simulink model "p4_system_arch_master"  (R2020a)
settings: Solver=VariableStepAuto  StartTime=0.0  StopTime=10.0  RelTol=1e-3
(part 4 of 11)

== system p4_system_arch_master/System 2 : Gearbox System/2.1 Torque Multiplication System/2.1.3 Gearset System 3 ==
  2.1.3.0.1 Pinion : ModelReference  ModelNameDialog=GearsetPinion  SimulationMode=Normal  ModelReferenceVersion=1.1
      settings: PortSchema="{\"entries\":[{\"content\":{\"headerSize\":38,\"margin\":15,\"minimumSpacing\":25,\"sides\":[{\"content\":{\"connectorIds\":[]},\"type\":\"ConnectorPlacement.EquallySpacedRectSide\",\"uuid\":\"a1de0a4a-4383-4256-97c8-b4b7017d79c3\"},{\"content\":{\"connectorIds\":[],\"side\":\"RIGHT\"},\"type\":\"ConnectorPlacement.EquallySpacedRectSide\",\"uuid\":\"b959f0e1-b665-4773-a9ab-23b80a79bba3\"},{\"content\":{\"connectorIds\":[],\"side\":\"TOP\"},\"type\":\"ConnectorPlacement.EquallySpacedRectSide\",\"uuid\":\"884e98bd-fa8a-4556-86a7-182eb6de8f96\"}]},\"type\":\"ConnectorPlacement.EquallySpacedConnector\",\"uuid\":\"31d5ce3f-6fbe-45a5-a872-1e90bd0aea01\"}],\"packageUris\":[\"http://schema.mathworks.com/mf0/Connector/19700101\"],\"version\":\"1.0\"}"
  2.1.3.0.2 Gear : Subsystem
      settings: PortSchema="{\"entries\":[{\"content\":{\"headerSize\":26,\"margin\":15,\"minimumSpacing\":25,\"sides\":[{\"content\":{\"connectorIds\":[]},\"type\":\"ConnectorPlacement.EquallySpacedRectSide\",\"uuid\":\"f8ee33a9-954f-44c6-a821-b5353f3278fa\"},{\"content\":{\"connectorIds\":[],\"side\":\"RIGHT\"},\"type\":\"ConnectorPlacement.EquallySpacedRectSide\",\"uuid\":\"385f1e4f-1c89-4afc-9c19-76a078cf90bc\"},{\"content\":{\"connectorIds\":[],\"side\":\"TOP\"},\"type\":\"ConnectorPlacement.EquallySpacedRectSide\",\"uuid\":\"fc91fa49-46f5-4ba7-960e-7bda5e0416d1\"}]},\"type\":\"ConnectorPlacement.EquallySpacedConnector\",\"uuid\":\"4bf08bc6-c7ce-47fb-af04-cd9d2b5f8092\"}],\"packageUris\":[\"http://schema.mathworks.com/mf0/Connector/19700101\"],\"version\":\"1.0\"}"

== system p4_system_arch_master/System 2 : Gearbox System/2.1 Torque Multiplication System/2.1.5 Bearings System ==
  Countershaft Bearings : Subsystem
      settings: PortSchema="{\"entries\":[{\"content\":{\"headerSize\":26,\"margin\":15,\"minimumSpacing\":25,\"sides\":[{\"content\":{\"connectorIds\":[]},\"type\":\"ConnectorPlacement.EquallySpacedRectSide\",\"uuid\":\"f8ee33a9-954f-44c6-a821-b5353f3278fa\"},{\"content\":{\"connectorIds\":[],\"side\":\"RIGHT\"},\"type\":\"ConnectorPlacement.EquallySpacedRectSide\",\"uuid\":\"385f1e4f-1c89-4afc-9c19-76a078cf90bc\"},{\"content\":{\"connectorIds\":[],\"side\":\"TOP\"},\"type\":\"ConnectorPlacement.EquallySpacedRectSide\",\"uuid\":\"fc91fa49-46f5-4ba7-960e-7bda5e0416d1\"}]},\"type\":\"ConnectorPlacement.EquallySpacedConnector\",\"uuid\":\"4bf08bc6-c7ce-47fb-af04-cd9d2b5f8092\"}],\"packageUris\":[\"http://schema.mathworks.com/mf0/Connector/19700101\"],\"version\":\"1.0\"}"
  Diff Bearings : Subsystem
      settings: PortSchema="{\"entries\":[{\"content\":{\"headerSize\":26,\"margin\":15,\"minimumSpacing\":25,\"sides\":[{\"content\":{\"connectorIds\":[]},\"type\":\"ConnectorPlacement.EquallySpacedRectSide\",\"uuid\":\"f8ee33a9-954f-44c6-a821-b5353f3278fa\"},{\"content\":{\"connectorIds\":[],\"side\":\"RIGHT\"},\"type\":\"ConnectorPlacement.EquallySpacedRectSide\",\"uuid\":\"385f1e4f-1c89-4afc-9c19-76a078cf90bc\"},{\"content\":{\"connectorIds\":[],\"side\":\"TOP\"},\"type\":\"ConnectorPlacement.EquallySpacedRectSide\",\"uuid\":\"fc91fa49-46f5-4ba7-960e-7bda5e0416d1\"}]},\"type\":\"ConnectorPlacement.EquallySpacedConnector\",\"uuid\":\"4bf08bc6-c7ce-47fb-af04-cd9d2b5f8092\"}],\"packageUris\":[\"http://schema.mathworks.com/mf0/Connector/19700101\"],\"version\":\"1.0\"}"
  Halfshaft Bearings : Subsystem
      settings: PortSchema="{\"entries\":[{\"content\":{\"headerSize\":26,\"margin\":15,\"minimumSpacing\":25,\"sides\":[{\"content\":{\"connectorIds\":[]},\"type\":\"ConnectorPlacement.EquallySpacedRectSide\",\"uuid\":\"f8ee33a9-954f-44c6-a821-b5353f3278fa\"},{\"content\":{\"connectorIds\":[],\"side\":\"RIGHT\"},\"type\":\"ConnectorPlacement.EquallySpacedRectSide\",\"uuid\":\"385f1e4f-1c89-4afc-9c19-76a078cf90bc\"},{\"content\":{\"connectorIds\":[],\"side\":\"TOP\"},\"type\":\"ConnectorPlacement.EquallySpacedRectSide\",\"uuid\":\"fc91fa49-46f5-4ba7-960e-7bda5e0416d1\"}]},\"type\":\"ConnectorPlacement.EquallySpacedConnector\",\"uuid\":\"4bf08bc6-c7ce-47fb-af04-cd9d2b5f8092\"}],\"packageUris\":[\"http://schema.mathworks.com/mf0/Connector/19700101\"],\"version\":\"1.0\"}"
  Input Shaft Bearings : Subsystem
      settings: PortSchema="{\"entries\":[{\"content\":{\"headerSize\":26,\"margin\":15,\"minimumSpacing\":25,\"sides\":[{\"content\":{\"connectorIds\":[]},\"type\":\"ConnectorPlacement.EquallySpacedRectSide\",\"uuid\":\"f8ee33a9-954f-44c6-a821-b5353f3278fa\"},{\"content\":{\"connectorIds\":[],\"side\":\"RIGHT\"},\"type\":\"ConnectorPlacement.EquallySpacedRectSide\",\"uuid\":\"385f1e4f-1c89-4afc-9c19-76a078cf90bc\"},{\"content\":{\"connectorIds\":[],\"side\":\"TOP\"},\"type\":\"ConnectorPlacement.EquallySpacedRectSide\",\"uuid\":\"fc91fa49-46f5-4ba7-960e-7bda5e0416d1\"}]},\"type\":\"ConnectorPlacement.EquallySpacedConnector\",\"uuid\":\"4bf08bc6-c7ce-47fb-af04-cd9d2b5f8092\"}],\"packageUris\":[\"http://schema.mathworks.com/mf0/Connector/19700101\"],\"version\":\"1.0\"}"

== system p4_system_arch_master/System 2 : Gearbox System/2.1 Torque Multiplication System/2.1.6 Axial Retention System  ==
  "2.1.6.0.1 Gs1 Bush " : Subsystem
      settings: PortSchema="{\"entries\":[{\"content\":{\"headerSize\":26,\"margin\":15,\"minimumSpacing\":25,\"sides\":[{\"content\":{\"connectorIds\":[]},\"type\":\"ConnectorPlacement.EquallySpacedRectSide\",\"uuid\":\"f8ee33a9-954f-44c6-a821-b5353f3278fa\"},{\"content\":{\"connectorIds\":[],\"side\":\"RIGHT\"},\"type\":\"ConnectorPlacement.EquallySpacedRectSide\",\"uuid\":\"385f1e4f-1c89-4afc-9c19-76a078cf90bc\"},{\"content\":{\"connectorIds\":[],\"side\":\"TOP\"},\"type\":\"ConnectorPlacement.EquallySpacedRectSide\",\"uuid\":\"fc91fa49-46f5-4ba7-960e-7bda5e0416d1\"}]},\"type\":\"ConnectorPlacement.EquallySpacedConnector\",\"uuid\":\"4bf08bc6-c7ce-47fb-af04-cd9d2b5f8092\"}],\"packageUris\":[\"http://schema.mathworks.com/mf0/Connector/19700101\"],\"version\":\"1.0\"}"
  2.1.6.0.2 Thrust Washer : Subsystem
      settings: PortSchema="{\"entries\":[{\"content\":{\"headerSize\":26,\"margin\":15,\"minimumSpacing\":25,\"sides\":[{\"content\":{\"connectorIds\":[]},\"type\":\"ConnectorPlacement.EquallySpacedRectSide\",\"uuid\":\"f8ee33a9-954f-44c6-a821-b5353f3278fa\"},{\"content\":{\"connectorIds\":[],\"side\":\"RIGHT\"},\"type\":\"ConnectorPlacement.EquallySpacedRectSide\",\"uuid\":\"385f1e4f-1c89-4afc-9c19-76a078cf90bc\"},{\"content\":{\"connectorIds\":[],\"side\":\"TOP\"},\"type\":\"ConnectorPlacement.EquallySpacedRectSide\",\"uuid\":\"fc91fa49-46f5-4ba7-960e-7bda5e0416d1\"}]},\"type\":\"ConnectorPlacement.EquallySpacedConnector\",\"uuid\":\"4bf08bc6-c7ce-47fb-af04-cd9d2b5f8092\"}],\"packageUris\":[\"http://schema.mathworks.com/mf0/Connector/19700101\"],\"version\":\"1.0\"}"
  2.1.6.0.3 Nb2 Washer : Subsystem
      settings: PortSchema="{\"entries\":[{\"content\":{\"headerSize\":26,\"margin\":15,\"minimumSpacing\":25,\"sides\":[{\"content\":{\"connectorIds\":[]},\"type\":\"ConnectorPlacement.EquallySpacedRectSide\",\"uuid\":\"f8ee33a9-954f-44c6-a821-b5353f3278fa\"},{\"content\":{\"connectorIds\":[],\"side\":\"RIGHT\"},\"type\":\"ConnectorPlacement.EquallySpacedRectSide\",\"uuid\":\"385f1e4f-1c89-4afc-9c19-76a078cf90bc\"},{\"content\":{\"connectorIds\":[],\"side\":\"TOP\"},\"type\":\"ConnectorPlacement.EquallySpacedRectSide\",\"uuid\":\"fc91fa49-46f5-4ba7-960e-7bda5e0416d1\"}]},\"type\":\"ConnectorPlacement.EquallySpacedConnector\",\"uuid\":\"4bf08bc6-c7ce-47fb-af04-cd9d2b5f8092\"}],\"packageUris\":[\"http://schema.mathworks.com/mf0/Connector/19700101\"],\"version\":\"1.0\"}"
  2.1.6.0.4 Gs3 Washer : Subsystem
      settings: PortSchema="{\"entries\":[{\"content\":{\"headerSize\":26,\"margin\":15,\"minimumSpacing\":25,\"sides\":[{\"content\":{\"connectorIds\":[]},\"type\":\"ConnectorPlacement.EquallySpacedRectSide\",\"uuid\":\"f8ee33a9-954f-44c6-a821-b5353f3278fa\"},{\"content\":{\"connectorIds\":[],\"side\":\"RIGHT\"},\"type\":\"ConnectorPlacement.EquallySpacedRectSide\",\"uuid\":\"385f1e4f-1c89-4afc-9c19-76a078cf90bc\"},{\"content\":{\"connectorIds\":[],\"side\":\"TOP\"},\"type\":\"ConnectorPlacement.EquallySpacedRectSide\",\"uuid\":\"fc91fa49-46f5-4ba7-960e-7bda5e0416d1\"}]},\"type\":\"ConnectorPlacement.EquallySpacedConnector\",\"uuid\":\"4bf08bc6-c7ce-47fb-af04-cd9d2b5f8092\"}],\"packageUris\":[\"http://schema.mathworks.com/mf0/Connector/19700101\"],\"version\":\"1.0\"}"
  2.1.6.0.7 B6_shim : Subsystem
      settings: PortSchema="{\"entries\":[{\"content\":{\"headerSize\":26,\"margin\":15,\"minimumSpacing\":25,\"sides\":[{\"content\":{\"connectorIds\":[]},\"type\":\"ConnectorPlacement.EquallySpacedRectSide\",\"uuid\":\"f8ee33a9-954f-44c6-a821-b5353f3278fa\"},{\"content\":{\"connectorIds\":[],\"side\":\"RIGHT\"},\"type\":\"ConnectorPlacement.EquallySpacedRectSide\",\"uuid\":\"385f1e4f-1c89-4afc-9c19-76a078cf90bc\"},{\"content\":{\"connectorIds\":[],\"side\":\"TOP\"},\"type\":\"ConnectorPlacement.EquallySpacedRectSide\",\"uuid\":\"fc91fa49-46f5-4ba7-960e-7bda5e0416d1\"}]},\"type\":\"ConnectorPlacement.EquallySpacedConnector\",\"uuid\":\"4bf08bc6-c7ce-47fb-af04-cd9d2b5f8092\"}],\"packageUris\":[\"http://schema.mathworks.com/mf0/Connector/19700101\"],\"version\":\"1.0\"}"
  2.1.6.0.8 Bolts : Subsystem
      settings: PortSchema="{\"entries\":[{\"content\":{\"headerSize\":26,\"margin\":15,\"minimumSpacing\":25,\"sides\":[{\"content\":{\"connectorIds\":[]},\"type\":\"ConnectorPlacement.EquallySpacedRectSide\",\"uuid\":\"f8ee33a9-954f-44c6-a821-b5353f3278fa\"},{\"content\":{\"connectorIds\":[],\"side\":\"RIGHT\"},\"type\":\"ConnectorPlacement.EquallySpacedRectSide\",\"uuid\":\"385f1e4f-1c89-4afc-9c19-76a078cf90bc\"},{\"content\":{\"connectorIds\":[],\"side\":\"TOP\"},\"type\":\"ConnectorPlacement.EquallySpacedRectSide\",\"uuid\":\"fc91fa49-46f5-4ba7-960e-7bda5e0416d1\"}]},\"type\":\"ConnectorPlacement.EquallySpacedConnector\",\"uuid\":\"4bf08bc6-c7ce-47fb-af04-cd9d2b5f8092\"}],\"packageUris\":[\"http://schema.mathworks.com/mf0/Connector/19700101\"],\"version\":\"1.0\"}"
  2.1.7.0.5 B2_shim : Subsystem
      settings: PortSchema="{\"entries\":[{\"content\":{\"headerSize\":26,\"margin\":15,\"minimumSpacing\":25,\"sides\":[{\"content\":{\"connectorIds\":[]},\"type\":\"ConnectorPlacement.EquallySpacedRectSide\",\"uuid\":\"f8ee33a9-954f-44c6-a821-b5353f3278fa\"},{\"content\":{\"connectorIds\":[],\"side\":\"RIGHT\"},\"type\":\"ConnectorPlacement.EquallySpacedRectSide\",\"uuid\":\"385f1e4f-1c89-4afc-9c19-76a078cf90bc\"},{\"content\":{\"connectorIds\":[],\"side\":\"TOP\"},\"type\":\"ConnectorPlacement.EquallySpacedRectSide\",\"uuid\":\"fc91fa49-46f5-4ba7-960e-7bda5e0416d1\"}]},\"type\":\"ConnectorPlacement.EquallySpacedConnector\",\"uuid\":\"4bf08bc6-c7ce-47fb-af04-cd9d2b5f8092\"}],\"packageUris\":[\"http://schema.mathworks.com/mf0/Connector/19700101\"],\"version\":\"1.0\"}"
  2.1.7.0.7 B4_shim : Subsystem
      settings: PortSchema="{\"entries\":[{\"content\":{\"headerSize\":26,\"margin\":15,\"minimumSpacing\":25,\"sides\":[{\"content\":{\"connectorIds\":[]},\"type\":\"ConnectorPlacement.EquallySpacedRectSide\",\"uuid\":\"f8ee33a9-954f-44c6-a821-b5353f3278fa\"},{\"content\":{\"connectorIds\":[],\"side\":\"RIGHT\"},\"type\":\"ConnectorPlacement.EquallySpacedRectSide\",\"uuid\":\"385f1e4f-1c89-4afc-9c19-76a078cf90bc\"},{\"content\":{\"connectorIds\":[],\"side\":\"TOP\"},\"type\":\"ConnectorPlacement.EquallySpacedRectSide\",\"uuid\":\"fc91fa49-46f5-4ba7-960e-7bda5e0416d1\"}]},\"type\":\"ConnectorPlacement.EquallySpacedConnector\",\"uuid\":\"4bf08bc6-c7ce-47fb-af04-cd9d2b5f8092\"}],\"packageUris\":[\"http://schema.mathworks.com/mf0/Connector/19700101\"],\"version\":\"1.0\"}"

== system p4_system_arch_master/System 2 : Gearbox System/2.1 Torque Multiplication System/Shaft System ==
  2.1.4.0.1 Countershaft S1 : Subsystem
      settings: PortSchema="{\"entries\":[{\"content\":{\"headerSize\":26,\"margin\":15,\"minimumSpacing\":25,\"sides\":[{\"content\":{\"connectorIds\":[]},\"type\":\"ConnectorPlacement.EquallySpacedRectSide\",\"uuid\":\"f8ee33a9-954f-44c6-a821-b5353f3278fa\"},{\"content\":{\"connectorIds\":[],\"side\":\"RIGHT\"},\"type\":\"ConnectorPlacement.EquallySpacedRectSide\",\"uuid\":\"385f1e4f-1c89-4afc-9c19-76a078cf90bc\"},{\"content\":{\"connectorIds\":[],\"side\":\"TOP\"},\"type\":\"ConnectorPlacement.EquallySpacedRectSide\",\"uuid\":\"fc91fa49-46f5-4ba7-960e-7bda5e0416d1\"}]},\"type\":\"ConnectorPlacement.EquallySpacedConnector\",\"uuid\":\"4bf08bc6-c7ce-47fb-af04-cd9d2b5f8092\"}],\"packageUris\":[\"http://schema.mathworks.com/mf0/Connector/19700101\"],\"version\":\"1.0\"}"
  "2.1.4.0.2 Input Shaft S2 " : Subsystem
      settings: PortSchema="{\"entries\":[{\"content\":{\"headerSize\":26,\"margin\":15,\"minimumSpacing\":25,\"sides\":[{\"content\":{\"connectorIds\":[]},\"type\":\"ConnectorPlacement.EquallySpacedRectSide\",\"uuid\":\"f8ee33a9-954f-44c6-a821-b5353f3278fa\"},{\"content\":{\"connectorIds\":[],\"side\":\"RIGHT\"},\"type\":\"ConnectorPlacement.EquallySpacedRectSide\",\"uuid\":\"385f1e4f-1c89-4afc-9c19-76a078cf90bc\"},{\"content\":{\"connectorIds\":[],\"side\":\"TOP\"},\"type\":\"ConnectorPlacement.EquallySpacedRectSide\",\"uuid\":\"fc91fa49-46f5-4ba7-960e-7bda5e0416d1\"}]},\"type\":\"ConnectorPlacement.EquallySpacedConnector\",\"uuid\":\"4bf08bc6-c7ce-47fb-af04-cd9d2b5f8092\"}],\"packageUris\":[\"http://schema.mathworks.com/mf0/Connector/19700101\"],\"version\":\"1.0\"}"

== system p4_system_arch_master/System 2 : Gearbox System/2.2 Gear Shifting System/Force Transfer System 2.2.2 ==
  "Fork Fixing System 2.2.2.3 " : Subsystem
      settings: PortSchema="{\"entries\":[{\"content\":{\"headerSize\":26,\"margin\":15,\"minimumSpacing\":25,\"sides\":[{\"content\":{\"connectorIds\":[]},\"type\":\"ConnectorPlacement.EquallySpacedRectSide\",\"uuid\":\"f8ee33a9-954f-44c6-a821-b5353f3278fa\"},{\"content\":{\"connectorIds\":[],\"side\":\"RIGHT\"},\"type\":\"ConnectorPlacement.EquallySpacedRectSide\",\"uuid\":\"385f1e4f-1c89-4afc-9c19-76a078cf90bc\"},{\"content\":{\"connectorIds\":[],\"side\":\"TOP\"},\"type\":\"ConnectorPlacement.EquallySpacedRectSide\",\"uuid\":\"fc91fa49-46f5-4ba7-960e-7bda5e0416d1\"}]},\"type\":\"ConnectorPlacement.EquallySpacedConnector\",\"uuid\":\"4bf08bc6-c7ce-47fb-af04-cd9d2b5f8092\"}],\"packageUris\":[\"http://schema.mathworks.com/mf0/Connector/19700101\"],\"version\":\"1.0\"}"
  "Gear Shift 1 System 2.2.2.1 " : Subsystem
      settings: PortSchema="{\"entries\":[{\"content\":{\"headerSize\":26,\"margin\":15,\"minimumSpacing\":25,\"sides\":[{\"content\":{\"connectorIds\":[]},\"type\":\"ConnectorPlacement.EquallySpacedRectSide\",\"uuid\":\"f8ee33a9-954f-44c6-a821-b5353f3278fa\"},{\"content\":{\"connectorIds\":[],\"side\":\"RIGHT\"},\"type\":\"ConnectorPlacement.EquallySpacedRectSide\",\"uuid\":\"385f1e4f-1c89-4afc-9c19-76a078cf90bc\"},{\"content\":{\"connectorIds\":[],\"side\":\"TOP\"},\"type\":\"ConnectorPlacement.EquallySpacedRectSide\",\"uuid\":\"fc91fa49-46f5-4ba7-960e-7bda5e0416d1\"}]},\"type\":\"ConnectorPlacement.EquallySpacedConnector\",\"uuid\":\"4bf08bc6-c7ce-47fb-af04-cd9d2b5f8092\"}],\"packageUris\":[\"http://schema.mathworks.com/mf0/Connector/19700101\"],\"version\":\"1.0\"}"
  "Gear Shift 2 System 2.2.2.2 " : Subsystem
      settings: PortSchema="{\"entries\":[{\"content\":{\"headerSize\":26,\"margin\":15,\"minimumSpacing\":25,\"sides\":[{\"content\":{\"connectorIds\":[]},\"type\":\"ConnectorPlacement.EquallySpacedRectSide\",\"uuid\":\"f8ee33a9-954f-44c6-a821-b5353f3278fa\"},{\"content\":{\"connectorIds\":[],\"side\":\"RIGHT\"},\"type\":\"ConnectorPlacement.EquallySpacedRectSide\",\"uuid\":\"385f1e4f-1c89-4afc-9c19-76a078cf90bc\"},{\"content\":{\"connectorIds\":[],\"side\":\"TOP\"},\"type\":\"ConnectorPlacement.EquallySpacedRectSide\",\"uuid\":\"fc91fa49-46f5-4ba7-960e-7bda5e0416d1\"}]},\"type\":\"ConnectorPlacement.EquallySpacedConnector\",\"uuid\":\"4bf08bc6-c7ce-47fb-af04-cd9d2b5f8092\"}],\"packageUris\":[\"http://schema.mathworks.com/mf0/Connector/19700101\"],\"version\":\"1.0\"}"

== system p4_system_arch_master/System 2 : Gearbox System/2.2 Gear Shifting System/Torque Transfer System 2.2.1  ==
  "Actuator Gearbox 2.2.1.1 " : Subsystem
      settings: PortSchema="{\"entries\":[{\"content\":{\"headerSize\":26,\"margin\":15,\"minimumSpacing\":25,\"sides\":[{\"content\":{\"connectorIds\":[]},\"type\":\"ConnectorPlacement.EquallySpacedRectSide\",\"uuid\":\"f8ee33a9-954f-44c6-a821-b5353f3278fa\"},{\"content\":{\"connectorIds\":[],\"side\":\"RIGHT\"},\"type\":\"ConnectorPlacement.EquallySpacedRectSide\",\"uuid\":\"385f1e4f-1c89-4afc-9c19-76a078cf90bc\"},{\"content\":{\"connectorIds\":[],\"side\":\"TOP\"},\"type\":\"ConnectorPlacement.EquallySpacedRectSide\",\"uuid\":\"fc91fa49-46f5-4ba7-960e-7bda5e0416d1\"}]},\"type\":\"ConnectorPlacement.EquallySpacedConnector\",\"uuid\":\"4bf08bc6-c7ce-47fb-af04-cd9d2b5f8092\"}],\"packageUris\":[\"http://schema.mathworks.com/mf0/Connector/19700101\"],\"version\":\"1.0\"}"
  "Drum Fixing System 2.2.1.3 " : Subsystem
      settings: PortSchema="{\"entries\":[{\"content\":{\"headerSize\":26,\"margin\":15,\"minimumSpacing\":25,\"sides\":[{\"content\":{\"connectorIds\":[]},\"type\":\"ConnectorPlacement.EquallySpacedRectSide\",\"uuid\":\"f8ee33a9-954f-44c6-a821-b5353f3278fa\"},{\"content\":{\"connectorIds\":[],\"side\":\"RIGHT\"},\"type\":\"ConnectorPlacement.EquallySpacedRectSide\",\"uuid\":\"385f1e4f-1c89-4afc-9c19-76a078cf90bc\"},{\"content\":{\"connectorIds\":[],\"side\":\"TOP\"},\"type\":\"ConnectorPlacement.EquallySpacedRectSide\",\"uuid\":\"fc91fa49-46f5-4ba7-960e-7bda5e0416d1\"}]},\"type\":\"ConnectorPlacement.EquallySpacedConnector\",\"uuid\":\"4bf08bc6-c7ce-47fb-af04-cd9d2b5f8092\"}],\"packageUris\":[\"http://schema.mathworks.com/mf0/Connector/19700101\"],\"version\":\"1.0\"}"
  "Torque to Force Translation 2.2.1.2 " : Subsystem
      settings: PortSchema="{\"entries\":[{\"content\":{\"headerSize\":26,\"margin\":15,\"minimumSpacing\":25,\"sides\":[{\"content\":{\"connectorIds\":[]},\"type\":\"ConnectorPlacement.EquallySpacedRectSide\",\"uuid\":\"f8ee33a9-954f-44c6-a821-b5353f3278fa\"},{\"content\":{\"connectorIds\":[],\"side\":\"RIGHT\"},\"type\":\"ConnectorPlacement.EquallySpacedRectSide\",\"uuid\":\"385f1e4f-1c89-4afc-9c19-76a078cf90bc\"},{\"content\":{\"connectorIds\":[],\"side\":\"TOP\"},\"type\":\"ConnectorPlacement.EquallySpacedRectSide\",\"uuid\":\"fc91fa49-46f5-4ba7-960e-7bda5e0416d1\"}]},\"type\":\"ConnectorPlacement.EquallySpacedConnector\",\"uuid\":\"4bf08bc6-c7ce-47fb-af04-cd9d2b5f8092\"}],\"packageUris\":[\"http://schema.mathworks.com/mf0/Connector/19700101\"],\"version\":\"1.0\"}"

== system p4_system_arch_master/System 3 : Torque Splitting System check /Differential System /Differential Body ==

== system p4_system_arch_master/System 3 : Torque Splitting System check /Differential System /Differential Pin ==

== system p4_system_arch_master/System 3 : Torque Splitting System check /Differential System /Gear Pinion 1 ==

== system p4_system_arch_master/System 3 : Torque Splitting System check /Differential System /Gear Pinion 2 ==

== system p4_system_arch_master/System 3 : Torque Splitting System check /Differential System /Gear Thrust Washer 1 ==

== system p4_system_arch_master/System 3 : Torque Splitting System check /Differential System /Gear Thrust Washer 2 ==

== system p4_system_arch_master/System 3 : Torque Splitting System check /Differential System /Gear Wheel 1 ==

== system p4_system_arch_master/System 3 : Torque Splitting System check /Differential System /Gear Wheel 2 ==

== system p4_system_arch_master/System 3 : Torque Splitting System check /Differential System /Pinion Thrust Washer 1 ==

== system p4_system_arch_master/System 3 : Torque Splitting System check /Differential System /Pinion Thrust Washer 2 ==

== system p4_system_arch_master/System 3 : Torque Splitting System check /Differential System /Roll Pin 1 ==

== system p4_system_arch_master/System 3 : Torque Splitting System check /Differential System /Roll Pin 2 ==

== system p4_system_arch_master/System 4 : Torque Transfer System/4.1 Link Shafts System/4.1.0.0.1 Link Shaft LH (LNKS1) ==

== system p4_system_arch_master/System 4 : Torque Transfer System/4.1 Link Shafts System/4.1.0.0.2 Link Shaft RH (LNKS2) ==

== system p4_system_arch_master/System 4 : Torque Transfer System/4.2 Support Brackets System/4.2.0.0.1 Support Bracket LH (SBR1) ==

== system p4_system_arch_master/System 4 : Torque Transfer System/4.2 Support Brackets System/4.2.0.0.2 Support Bracket RH (SBR2) ==

== system p4_system_arch_master/System 4 : Torque Transfer System/4.3 Bearing, Fixing & Sealing System/4.3.0.0.1 Bearing 7 (B7) ==

== system p4_system_arch_master/System 4 : Torque Transfer System/4.3 Bearing, Fixing & Sealing System/4.3.0.0.10 Tulip Snap Ring RH (TSR2) ==

== system p4_system_arch_master/System 4 : Torque Transfer System/4.3 Bearing, Fixing & Sealing System/4.3.0.0.11 Differential Snap Ring LH (DSR1) ==

== system p4_system_arch_master/System 4 : Torque Transfer System/4.3 Bearing, Fixing & Sealing System/4.3.0.0.12 Differential Snap Ring RH (DSR2) ==

== system p4_system_arch_master/System 4 : Torque Transfer System/4.3 Bearing, Fixing & Sealing System/4.3.0.0.13 Support Bracket LH Bolts ==
  Support Bracket LH Bolt {1..4} (4 alike) : ModelReference  ModelNameDialog=M6x30  SimulationMode=Normal  ModelReferenceVersion=1.1
      settings: PortSchema="{\"entries\":[{\"content\":{\"headerSize\":38,\"margin\":15,\"minimumSpacing\":25,\"sides\":[{\"content\":{\"connectorIds\":[]},\"type\":\"ConnectorPlacement.EquallySpacedRectSide\",\"uuid\":\"a1de0a4a-4383-4256-97c8-b4b7017d79c3\"},{\"content\":{\"connectorIds\":[],\"side\":\"RIGHT\"},\"type\":\"ConnectorPlacement.EquallySpacedRectSide\",\"uuid\":\"b959f0e1-b665-4773-a9ab-23b80a79bba3\"},{\"content\":{\"connectorIds\":[],\"side\":\"TOP\"},\"type\":\"ConnectorPlacement.EquallySpacedRectSide\",\"uuid\":\"884e98bd-fa8a-4556-86a7-182eb6de8f96\"}]},\"type\":\"ConnectorPlacement.EquallySpacedConnector\",\"uuid\":\"31d5ce3f-6fbe-45a5-a872-1e90bd0aea01\"}],\"packageUris\":[\"http://schema.mathworks.com/mf0/Connector/19700101\"],\"version\":\"1.0\"}"

== system p4_system_arch_master/System 4 : Torque Transfer System/4.3 Bearing, Fixing & Sealing System/4.3.0.0.14 Support Bracket RH Bolts ==
  Support Bracket RH Bolt {1..4} (4 alike) : ModelReference  ModelNameDialog=M6x30  SimulationMode=Normal  ModelReferenceVersion=1.1
      settings: PortSchema="{\"entries\":[{\"content\":{\"headerSize\":38,\"margin\":15,\"minimumSpacing\":25,\"sides\":[{\"content\":{\"connectorIds\":[]},\"type\":\"ConnectorPlacement.EquallySpacedRectSide\",\"uuid\":\"a1de0a4a-4383-4256-97c8-b4b7017d79c3\"},{\"content\":{\"connectorIds\":[],\"side\":\"RIGHT\"},\"type\":\"ConnectorPlacement.EquallySpacedRectSide\",\"uuid\":\"b959f0e1-b665-4773-a9ab-23b80a79bba3\"},{\"content\":{\"connectorIds\":[],\"side\":\"TOP\"},\"type\":\"ConnectorPlacement.EquallySpacedRectSide\",\"uuid\":\"884e98bd-fa8a-4556-86a7-182eb6de8f96\"}]},\"type\":\"ConnectorPlacement.EquallySpacedConnector\",\"uuid\":\"31d5ce3f-6fbe-45a5-a872-1e90bd0aea01\"}],\"packageUris\":[\"http://schema.mathworks.com/mf0/Connector/19700101\"],\"version\":\"1.0\"}"

== system p4_system_arch_master/System 4 : Torque Transfer System/4.3 Bearing, Fixing & Sealing System/4.3.0.0.2 Bearing 8 (B8) ==

== system p4_system_arch_master/System 4 : Torque Transfer System/4.3 Bearing, Fixing & Sealing System/4.3.0.0.3 Bearing External Circlip LH (BEC1) ==

== system p4_system_arch_master/System 4 : Torque Transfer System/4.3 Bearing, Fixing & Sealing System/4.3.0.0.4 Bearing External Circlip RH (BEC2) ==

== system p4_system_arch_master/System 4 : Torque Transfer System/4.3 Bearing, Fixing & Sealing System/4.3.0.0.5 Bearing Internal Circlip LH (BIC1) ==

== system p4_system_arch_master/System 4 : Torque Transfer System/4.3 Bearing, Fixing & Sealing System/4.3.0.0.6 Bearing Internal Circlip RH (BIC2) ==

== system p4_system_arch_master/System 4 : Torque Transfer System/4.3 Bearing, Fixing & Sealing System/4.3.0.0.7 O-Ring LH (OR1) ==

== system p4_system_arch_master/System 4 : Torque Transfer System/4.3 Bearing, Fixing & Sealing System/4.3.0.0.8 O-Ring RH (OR2) ==

== system p4_system_arch_master/System 4 : Torque Transfer System/4.3 Bearing, Fixing & Sealing System/4.3.0.0.9 Tulip Snap Ring LH (TSR1) ==

== system p4_system_arch_master/System 5 : Enclosure and Sealing System X/5.1 Component Enclosure System/5.1.2 RH Gearbox, Motor and Inverter Enclosure System ==
  "5.1.2.0.1 RH Gearbox, Motor and Inverter Casing" : Subsystem
      settings: PortSchema="{\"entries\":[{\"content\":{\"headerSize\":26,\"margin\":15,\"minimumSpacing\":25,\"sides\":[{\"content\":{\"connectorIds\":[]},\"type\":\"ConnectorPlacement.EquallySpacedRectSide\",\"uuid\":\"f8ee33a9-954f-44c6-a821-b5353f3278fa\"},{\"content\":{\"connectorIds\":[],\"side\":\"RIGHT\"},\"type\":\"ConnectorPlacement.EquallySpacedRectSide\",\"uuid\":\"385f1e4f-1c89-4afc-9c19-76a078cf90bc\"},{\"content\":{\"connectorIds\":[],\"side\":\"TOP\"},\"type\":\"ConnectorPlacement.EquallySpacedRectSide\",\"uuid\":\"fc91fa49-46f5-4ba7-960e-7bda5e0416d1\"}]},\"type\":\"ConnectorPlacement.EquallySpacedConnector\",\"uuid\":\"4bf08bc6-c7ce-47fb-af04-cd9d2b5f8092\"}],\"packageUris\":[\"http://schema.mathworks.com/mf0/Connector/19700101\"],\"version\":\"1.0\"}"
  5.1.2.0.2 NDE Motor Cover : Subsystem
      settings: PortSchema="{\"entries\":[{\"content\":{\"headerSize\":26,\"margin\":15,\"minimumSpacing\":25,\"sides\":[{\"content\":{\"connectorIds\":[]},\"type\":\"ConnectorPlacement.EquallySpacedRectSide\",\"uuid\":\"f8ee33a9-954f-44c6-a821-b5353f3278fa\"},{\"content\":{\"connectorIds\":[],\"side\":\"RIGHT\"},\"type\":\"ConnectorPlacement.EquallySpacedRectSide\",\"uuid\":\"385f1e4f-1c89-4afc-9c19-76a078cf90bc\"},{\"content\":{\"connectorIds\":[],\"side\":\"TOP\"},\"type\":\"ConnectorPlacement.EquallySpacedRectSide\",\"uuid\":\"fc91fa49-46f5-4ba7-960e-7bda5e0416d1\"}]},\"type\":\"ConnectorPlacement.EquallySpacedConnector\",\"uuid\":\"4bf08bc6-c7ce-47fb-af04-cd9d2b5f8092\"}],\"packageUris\":[\"http://schema.mathworks.com/mf0/Connector/19700101\"],\"version\":\"1.0\"}"
  5.1.2.0.3 Resolver Cover : Subsystem
      settings: PortSchema="{\"entries\":[{\"content\":{\"headerSize\":26,\"margin\":15,\"minimumSpacing\":25,\"sides\":[{\"content\":{\"connectorIds\":[]},\"type\":\"ConnectorPlacement.EquallySpacedRectSide\",\"uuid\":\"f8ee33a9-954f-44c6-a821-b5353f3278fa\"},{\"content\":{\"connectorIds\":[],\"side\":\"RIGHT\"},\"type\":\"ConnectorPlacement.EquallySpacedRectSide\",\"uuid\":\"385f1e4f-1c89-4afc-9c19-76a078cf90bc\"},{\"content\":{\"connectorIds\":[],\"side\":\"TOP\"},\"type\":\"ConnectorPlacement.EquallySpacedRectSide\",\"uuid\":\"fc91fa49-46f5-4ba7-960e-7bda5e0416d1\"}]},\"type\":\"ConnectorPlacement.EquallySpacedConnector\",\"uuid\":\"4bf08bc6-c7ce-47fb-af04-cd9d2b5f8092\"}],\"packageUris\":[\"http://schema.mathworks.com/mf0/Connector/19700101\"],\"version\":\"1.0\"}"
  5.1.2.0.4 Top Inverter Cover : Subsystem
      settings: PortSchema="{\"entries\":[{\"content\":{\"headerSize\":26,\"margin\":15,\"minimumSpacing\":25,\"sides\":[{\"content\":{\"connectorIds\":[]},\"type\":\"ConnectorPlacement.EquallySpacedRectSide\",\"uuid\":\"f8ee33a9-954f-44c6-a821-b5353f3278fa\"},{\"content\":{\"connectorIds\":[],\"side\":\"RIGHT\"},\"type\":\"ConnectorPlacement.EquallySpacedRectSide\",\"uuid\":\"385f1e4f-1c89-4afc-9c19-76a078cf90bc\"},{\"content\":{\"connectorIds\":[],\"side\":\"TOP\"},\"type\":\"ConnectorPlacement.EquallySpacedRectSide\",\"uuid\":\"fc91fa49-46f5-4ba7-960e-7bda5e0416d1\"}]},\"type\":\"ConnectorPlacement.EquallySpacedConnector\",\"uuid\":\"4bf08bc6-c7ce-47fb-af04-cd9d2b5f8092\"}],\"packageUris\":[\"http://schema.mathworks.com/mf0/Connector/19700101\"],\"version\":\"1.0\"}"

== system p4_system_arch_master/System 5 : Enclosure and Sealing System X/5.1 Component Enclosure System/LH Gearbox Enclosure ==

== system p4_system_arch_master/System 5 : Enclosure and Sealing System X/5.2 Sealing System/5.2.1 Rotary Seals System ==
  5.2.1.0.1 Differential rotary seal LH (SL1) : Subsystem
      settings: PortSchema="{\"entries\":[{\"content\":{\"headerSize\":26,\"margin\":15,\"minimumSpacing\":25,\"sides\":[{\"content\":{\"connectorIds\":[]},\"type\":\"ConnectorPlacement.EquallySpacedRectSide\",\"uuid\":\"f8ee33a9-954f-44c6-a821-b5353f3278fa\"},{\"content\":{\"connectorIds\":[],\"side\":\"RIGHT\"},\"type\":\"ConnectorPlacement.EquallySpacedRectSide\",\"uuid\":\"385f1e4f-1c89-4afc-9c19-76a078cf90bc\"},{\"content\":{\"connectorIds\":[],\"side\":\"TOP\"},\"type\":\"ConnectorPlacement.EquallySpacedRectSide\",\"uuid\":\"fc91fa49-46f5-4ba7-960e-7bda5e0416d1\"}]},\"type\":\"ConnectorPlacement.EquallySpacedConnector\",\"uuid\":\"4bf08bc6-c7ce-47fb-af04-cd9d2b5f8092\"}],\"packageUris\":[\"http://schema.mathworks.com/mf0/Connector/19700101\"],\"version\":\"1.0\"}"
  5.2.1.0.2 Barrel Cam Rotary Seal (SL4) : Subsystem
      settings: PortSchema="{\"entries\":[{\"content\":{\"headerSize\":26,\"margin\":15,\"minimumSpacing\":25,\"sides\":[{\"content\":{\"connectorIds\":[]},\"type\":\"ConnectorPlacement.EquallySpacedRectSide\",\"uuid\":\"f8ee33a9-954f-44c6-a821-b5353f3278fa\"},{\"content\":{\"connectorIds\":[],\"side\":\"RIGHT\"},\"type\":\"ConnectorPlacement.EquallySpacedRectSide\",\"uuid\":\"385f1e4f-1c89-4afc-9c19-76a078cf90bc\"},{\"content\":{\"connectorIds\":[],\"side\":\"TOP\"},\"type\":\"ConnectorPlacement.EquallySpacedRectSide\",\"uuid\":\"fc91fa49-46f5-4ba7-960e-7bda5e0416d1\"}]},\"type\":\"ConnectorPlacement.EquallySpacedConnector\",\"uuid\":\"4bf08bc6-c7ce-47fb-af04-cd9d2b5f8092\"}],\"packageUris\":[\"http://schema.mathworks.com/mf0/Connector/19700101\"],\"version\":\"1.0\"}"
  5.2.1.0.3 Differential rotary seal RH (SL2) : Subsystem
      settings: PortSchema="{\"entries\":[{\"content\":{\"headerSize\":26,\"margin\":15,\"minimumSpacing\":25,\"sides\":[{\"content\":{\"connectorIds\":[]},\"type\":\"ConnectorPlacement.EquallySpacedRectSide\",\"uuid\":\"f8ee33a9-954f-44c6-a821-b5353f3278fa\"},{\"content\":{\"connectorIds\":[],\"side\":\"RIGHT\"},\"type\":\"ConnectorPlacement.EquallySpacedRectSide\",\"uuid\":\"385f1e4f-1c89-4afc-9c19-76a078cf90bc\"},{\"content\":{\"connectorIds\":[],\"side\":\"TOP\"},\"type\":\"ConnectorPlacement.EquallySpacedRectSide\",\"uuid\":\"fc91fa49-46f5-4ba7-960e-7bda5e0416d1\"}]},\"type\":\"ConnectorPlacement.EquallySpacedConnector\",\"uuid\":\"4bf08bc6-c7ce-47fb-af04-cd9d2b5f8092\"}],\"packageUris\":[\"http://schema.mathworks.com/mf0/Connector/19700101\"],\"version\":\"1.0\"}"
  5.2.1.0.4 Input shaft rotary seal (SL3) : Subsystem
      settings: PortSchema="{\"entries\":[{\"content\":{\"headerSize\":26,\"margin\":15,\"minimumSpacing\":25,\"sides\":[{\"content\":{\"connectorIds\":[]},\"type\":\"ConnectorPlacement.EquallySpacedRectSide\",\"uuid\":\"f8ee33a9-954f-44c6-a821-b5353f3278fa\"},{\"content\":{\"connectorIds\":[],\"side\":\"RIGHT\"},\"type\":\"ConnectorPlacement.EquallySpacedRectSide\",\"uuid\":\"385f1e4f-1c89-4afc-9c19-76a078cf90bc\"},{\"content\":{\"connectorIds\":[],\"side\":\"TOP\"},\"type\":\"ConnectorPlacement.EquallySpacedRectSide\",\"uuid\":\"fc91fa49-46f5-4ba7-960e-7bda5e0416d1\"}]},\"type\":\"ConnectorPlacement.EquallySpacedConnector\",\"uuid\":\"4bf08bc6-c7ce-47fb-af04-cd9d2b5f8092\"}],\"packageUris\":[\"http://schema.mathworks.com/mf0/Connector/19700101\"],\"version\":\"1.0\"}"

== system p4_system_arch_master/System 5 : Enclosure and Sealing System X/5.2 Sealing System/5.2.2 Static Seals System ==
  5.2.2.1 Static - Flat Surface Sealing System : Subsystem
      settings: PortSchema="{\"entries\":[{\"content\":{\"headerSize\":26,\"margin\":15,\"minimumSpacing\":25,\"sides\":[{\"content\":{\"connectorIds\":[]},\"type\":\"ConnectorPlacement.EquallySpacedRectSide\",\"uuid\":\"f8ee33a9-954f-44c6-a821-b5353f3278fa\"},{\"content\":{\"connectorIds\":[],\"side\":\"RIGHT\"},\"type\":\"ConnectorPlacement.EquallySpacedRectSide\",\"uuid\":\"385f1e4f-1c89-4afc-9c19-76a078cf90bc\"},{\"content\":{\"connectorIds\":[],\"side\":\"TOP\"},\"type\":\"ConnectorPlacement.EquallySpacedRectSide\",\"uuid\":\"fc91fa49-46f5-4ba7-960e-7bda5e0416d1\"}]},\"type\":\"ConnectorPlacement.EquallySpacedConnector\",\"uuid\":\"4bf08bc6-c7ce-47fb-af04-cd9d2b5f8092\"}],\"packageUris\":[\"http://schema.mathworks.com/mf0/Connector/19700101\"],\"version\":\"1.0\"}"
  5.2.2.2 Static O-Rings & Washers : Subsystem
      settings: PortSchema="{\"entries\":[{\"content\":{\"headerSize\":26,\"margin\":15,\"minimumSpacing\":25,\"sides\":[{\"content\":{\"connectorIds\":[]},\"type\":\"ConnectorPlacement.EquallySpacedRectSide\",\"uuid\":\"f8ee33a9-954f-44c6-a821-b5353f3278fa\"},{\"content\":{\"connectorIds\":[],\"side\":\"RIGHT\"},\"type\":\"ConnectorPlacement.EquallySpacedRectSide\",\"uuid\":\"385f1e4f-1c89-4afc-9c19-76a078cf90bc\"},{\"content\":{\"connectorIds\":[],\"side\":\"TOP\"},\"type\":\"ConnectorPlacement.EquallySpacedRectSide\",\"uuid\":\"fc91fa49-46f5-4ba7-960e-7bda5e0416d1\"}]},\"type\":\"ConnectorPlacement.EquallySpacedConnector\",\"uuid\":\"4bf08bc6-c7ce-47fb-af04-cd9d2b5f8092\"}],\"packageUris\":[\"http://schema.mathworks.com/mf0/Connector/19700101\"],\"version\":\"1.0\"}"

== system p4_system_arch_master/System 5 : Enclosure and Sealing System X/5.3 Component Enclosure Peripherals X/5.3.1 Fixing, Indexation and Labeling System ==
  5.3.1.1 Gearbox Enclosures Fixing System : Subsystem
      settings: PortSchema="{\"entries\":[{\"content\":{\"headerSize\":26,\"margin\":15,\"minimumSpacing\":25,\"sides\":[{\"content\":{\"connectorIds\":[]},\"type\":\"ConnectorPlacement.EquallySpacedRectSide\",\"uuid\":\"f8ee33a9-954f-44c6-a821-b5353f3278fa\"},{\"content\":{\"connectorIds\":[],\"side\":\"RIGHT\"},\"type\":\"ConnectorPlacement.EquallySpacedRectSide\",\"uuid\":\"385f1e4f-1c89-4afc-9c19-76a078cf90bc\"},{\"content\":{\"connectorIds\":[],\"side\":\"TOP\"},\"type\":\"ConnectorPlacement.EquallySpacedRectSide\",\"uuid\":\"fc91fa49-46f5-4ba7-960e-7bda5e0416d1\"}]},\"type\":\"ConnectorPlacement.EquallySpacedConnector\",\"uuid\":\"4bf08bc6-c7ce-47fb-af04-cd9d2b5f8092\"}],\"packageUris\":[\"http://schema.mathworks.com/mf0/Connector/19700101\"],\"version\":\"1.0\"}"
  5.3.1.2 Gearbox Enclosures Indexation System : Subsystem
      settings: PortSchema="{\"entries\":[{\"content\":{\"headerSize\":26,\"margin\":15,\"minimumSpacing\":25,\"sides\":[{\"content\":{\"connectorIds\":[]},\"type\":\"ConnectorPlacement.EquallySpacedRectSide\",\"uuid\":\"f8ee33a9-954f-44c6-a821-b5353f3278fa\"},{\"content\":{\"connectorIds\":[],\"side\":\"RIGHT\"},\"type\":\"ConnectorPlacement.EquallySpacedRectSide\",\"uuid\":\"385f1e4f-1c89-4afc-9c19-76a078cf90bc\"},{\"content\":{\"connectorIds\":[],\"side\":\"TOP\"},\"type\":\"ConnectorPlacement.EquallySpacedRectSide\",\"uuid\":\"fc91fa49-46f5-4ba7-960e-7bda5e0416d1\"}]},\"type\":\"ConnectorPlacement.EquallySpacedConnector\",\"uuid\":\"4bf08bc6-c7ce-47fb-af04-cd9d2b5f8092\"}],\"packageUris\":[\"http://schema.mathworks.com/mf0/Connector/19700101\"],\"version\":\"1.0\"}"

== system p4_system_arch_master/System 5 : Enclosure and Sealing System X/5.3 Component Enclosure Peripherals X/5.3.2 Lubrication and Cooling Peripherals ==
  5.3.2.1 Lubrication System Peripherals : Subsystem
      settings: PortSchema="{\"entries\":[{\"content\":{\"headerSize\":26,\"margin\":15,\"minimumSpacing\":25,\"sides\":[{\"content\":{\"connectorIds\":[]},\"type\":\"ConnectorPlacement.EquallySpacedRectSide\",\"uuid\":\"f8ee33a9-954f-44c6-a821-b5353f3278fa\"},{\"content\":{\"connectorIds\":[],\"side\":\"RIGHT\"},\"type\":\"ConnectorPlacement.EquallySpacedRectSide\",\"uuid\":\"385f1e4f-1c89-4afc-9c19-76a078cf90bc\"},{\"content\":{\"connectorIds\":[],\"side\":\"TOP\"},\"type\":\"ConnectorPlacement.EquallySpacedRectSide\",\"uuid\":\"fc91fa49-46f5-4ba7-960e-7bda5e0416d1\"}]},\"type\":\"ConnectorPlacement.EquallySpacedConnector\",\"uuid\":\"4bf08bc6-c7ce-47fb-af04-cd9d2b5f8092\"}],\"packageUris\":[\"http://schema.mathworks.com/mf0/Connector/19700101\"],\"version\":\"1.0\"}"
  5.3.2.3 Gearbox Venting & Aerating System : Subsystem
      settings: PortSchema="{\"entries\":[{\"content\":{\"headerSize\":26,\"margin\":15,\"minimumSpacing\":25,\"sides\":[{\"content\":{\"connectorIds\":[]},\"type\":\"ConnectorPlacement.EquallySpacedRectSide\",\"uuid\":\"f8ee33a9-954f-44c6-a821-b5353f3278fa\"},{\"content\":{\"connectorIds\":[],\"side\":\"RIGHT\"},\"type\":\"ConnectorPlacement.EquallySpacedRectSide\",\"uuid\":\"385f1e4f-1c89-4afc-9c19-76a078cf90bc\"},{\"content\":{\"connectorIds\":[],\"side\":\"TOP\"},\"type\":\"ConnectorPlacement.EquallySpacedRectSide\",\"uuid\":\"fc91fa49-46f5-4ba7-960e-7bda5e0416d1\"}]},\"type\":\"ConnectorPlacement.EquallySpacedConnector\",\"uuid\":\"4bf08bc6-c7ce-47fb-af04-cd9d2b5f8092\"}],\"packageUris\":[\"http://schema.mathworks.com/mf0/Connector/19700101\"],\"version\":\"1.0\"}"
  5.3.2.4 Cooling Peripherals : Subsystem
      settings: PortSchema="{\"entries\":[{\"content\":{\"headerSize\":26,\"margin\":15,\"minimumSpacing\":25,\"sides\":[{\"content\":{\"connectorIds\":[]},\"type\":\"ConnectorPlacement.EquallySpacedRectSide\",\"uuid\":\"f8ee33a9-954f-44c6-a821-b5353f3278fa\"},{\"content\":{\"connectorIds\":[],\"side\":\"RIGHT\"},\"type\":\"ConnectorPlacement.EquallySpacedRectSide\",\"uuid\":\"385f1e4f-1c89-4afc-9c19-76a078cf90bc\"},{\"content\":{\"connectorIds\":[],\"side\":\"TOP\"},\"type\":\"ConnectorPlacement.EquallySpacedRectSide\",\"uuid\":\"fc91fa49-46f5-4ba7-960e-7bda5e0416d1\"}]},\"type\":\"ConnectorPlacement.EquallySpacedConnector\",\"uuid\":\"4bf08bc6-c7ce-47fb-af04-cd9d2b5f8092\"}],\"packageUris\":[\"http://schema.mathworks.com/mf0/Connector/19700101\"],\"version\":\"1.0\"}"

== system p4_system_arch_master/System 5 : Enclosure and Sealing System X/5.3 Component Enclosure Peripherals X/5.3.3 Cable Fixing System ==
  5.3.3.0.1 LV cables clips : Subsystem
      settings: PortSchema="{\"entries\":[{\"content\":{\"headerSize\":26,\"margin\":15,\"minimumSpacing\":25,\"sides\":[{\"content\":{\"connectorIds\":[]},\"type\":\"ConnectorPlacement.EquallySpacedRectSide\",\"uuid\":\"f8ee33a9-954f-44c6-a821-b5353f3278fa\"},{\"content\":{\"connectorIds\":[],\"side\":\"RIGHT\"},\"type\":\"ConnectorPlacement.EquallySpacedRectSide\",\"uuid\":\"385f1e4f-1c89-4afc-9c19-76a078cf90bc\"},{\"content\":{\"connectorIds\":[],\"side\":\"TOP\"},\"type\":\"ConnectorPlacement.EquallySpacedRectSide\",\"uuid\":\"fc91fa49-46f5-4ba7-960e-7bda5e0416d1\"}]},\"type\":\"ConnectorPlacement.EquallySpacedConnector\",\"uuid\":\"4bf08bc6-c7ce-47fb-af04-cd9d2b5f8092\"}],\"packageUris\":[\"http://schema.mathworks.com/mf0/Connector/19700101\"],\"version\":\"1.0\"}"

== system p4_system_arch_master/System 6 : Sensor and Actuation System/6.1 Sensor System /6.1.1 Gearbox Output Speed Measuring SubSystem  ==
  6.1.1.0.1 Gearbox Output Speed Measurement Subsystem - body : Subsystem
      settings: PortSchema="{\"entries\":[{\"content\":{\"headerSize\":26,\"margin\":15,\"minimumSpacing\":25,\"sides\":[{\"content\":{\"connectorIds\":[]},\"type\":\"ConnectorPlacement.EquallySpacedRectSide\",\"uuid\":\"f8ee33a9-954f-44c6-a821-b5353f3278fa\"},{\"content\":{\"connectorIds\":[],\"side\":\"RIGHT\"},\"type\":\"ConnectorPlacement.EquallySpacedRectSide\",\"uuid\":\"385f1e4f-1c89-4afc-9c19-76a078cf90bc\"},{\"content\":{\"connectorIds\":[],\"side\":\"TOP\"},\"type\":\"ConnectorPlacement.EquallySpacedRectSide\",\"uuid\":\"fc91fa49-46f5-4ba7-960e-7bda5e0416d1\"}]},\"type\":\"ConnectorPlacement.EquallySpacedConnector\",\"uuid\":\"4bf08bc6-c7ce-47fb-af04-cd9d2b5f8092\"}],\"packageUris\":[\"http://schema.mathworks.com/mf0/Connector/19700101\"],\"version\":\"1.0\"}"
  "6.1.1.0.2  Gearbox Output Speed Measurement Subsystem - O-ring " : Subsystem
      settings: PortSchema="{\"entries\":[{\"content\":{\"headerSize\":26,\"margin\":15,\"minimumSpacing\":25,\"sides\":[{\"content\":{\"connectorIds\":[]},\"type\":\"ConnectorPlacement.EquallySpacedRectSide\",\"uuid\":\"f8ee33a9-954f-44c6-a821-b5353f3278fa\"},{\"content\":{\"connectorIds\":[],\"side\":\"RIGHT\"},\"type\":\"ConnectorPlacement.EquallySpacedRectSide\",\"uuid\":\"385f1e4f-1c89-4afc-9c19-76a078cf90bc\"},{\"content\":{\"connectorIds\":[],\"side\":\"TOP\"},\"type\":\"ConnectorPlacement.EquallySpacedRectSide\",\"uuid\":\"fc91fa49-46f5-4ba7-960e-7bda5e0416d1\"}]},\"type\":\"ConnectorPlacement.EquallySpacedConnector\",\"uuid\":\"4bf08bc6-c7ce-47fb-af04-cd9d2b5f8092\"}],\"packageUris\":[\"http://schema.mathworks.com/mf0/Connector/19700101\"],\"version\":\"1.0\"}"

== system p4_system_arch_master/System 6 : Sensor and Actuation System/6.1 Sensor System /6.1.2 Gearbox Input Speed Measurement Subsystem ==
  6.1.2.0.1 Gearbox Input Speed Measurement Subsystem - body : Subsystem
      settings: PortSchema="{\"entries\":[{\"content\":{\"headerSize\":26,\"margin\":15,\"minimumSpacing\":25,\"sides\":[{\"content\":{\"connectorIds\":[]},\"type\":\"ConnectorPlacement.EquallySpacedRectSide\",\"uuid\":\"f8ee33a9-954f-44c6-a821-b5353f3278fa\"},{\"content\":{\"connectorIds\":[],\"side\":\"RIGHT\"},\"type\":\"ConnectorPlacement.EquallySpacedRectSide\",\"uuid\":\"385f1e4f-1c89-4afc-9c19-76a078cf90bc\"},{\"content\":{\"connectorIds\":[],\"side\":\"TOP\"},\"type\":\"ConnectorPlacement.EquallySpacedRectSide\",\"uuid\":\"fc91fa49-46f5-4ba7-960e-7bda5e0416d1\"}]},\"type\":\"ConnectorPlacement.EquallySpacedConnector\",\"uuid\":\"4bf08bc6-c7ce-47fb-af04-cd9d2b5f8092\"}],\"packageUris\":[\"http://schema.mathworks.com/mf0/Connector/19700101\"],\"version\":\"1.0\"}"
  "6.1.2.0.2  Gearbox Input Speed Measurement Subsystem - O-ring " : Subsystem
      settings: PortSchema="{\"entries\":[{\"content\":{\"headerSize\":26,\"margin\":15,\"minimumSpacing\":25,\"sides\":[{\"content\":{\"connectorIds\":[]},\"type\":\"ConnectorPlacement.EquallySpacedRectSide\",\"uuid\":\"f8ee33a9-954f-44c6-a821-b5353f3278fa\"},{\"content\":{\"connectorIds\":[],\"side\":\"RIGHT\"},\"type\":\"ConnectorPlacement.EquallySpacedRectSide\",\"uuid\":\"385f1e4f-1c89-4afc-9c19-76a078cf90bc\"},{\"content\":{\"connectorIds\":[],\"side\":\"TOP\"},\"type\":\"ConnectorPlacement.EquallySpacedRectSide\",\"uuid\":\"fc91fa49-46f5-4ba7-960e-7bda5e0416d1\"}]},\"type\":\"ConnectorPlacement.EquallySpacedConnector\",\"uuid\":\"4bf08bc6-c7ce-47fb-af04-cd9d2b5f8092\"}],\"packageUris\":[\"http://schema.mathworks.com/mf0/Connector/19700101\"],\"version\":\"1.0\"}"

== system p4_system_arch_master/System 6 : Sensor and Actuation System/6.1 Sensor System /6.1.3 Gearbox Temperature Measurement SubSystem  ==
  6.1.3.0.1 Gearbox Temperature Measurement Subsystem - body : Subsystem
      settings: PortSchema="{\"entries\":[{\"content\":{\"headerSize\":26,\"margin\":15,\"minimumSpacing\":25,\"sides\":[{\"content\":{\"connectorIds\":[]},\"type\":\"ConnectorPlacement.EquallySpacedRectSide\",\"uuid\":\"f8ee33a9-954f-44c6-a821-b5353f3278fa\"},{\"content\":{\"connectorIds\":[],\"side\":\"RIGHT\"},\"type\":\"ConnectorPlacement.EquallySpacedRectSide\",\"uuid\":\"385f1e4f-1c89-4afc-9c19-76a078cf90bc\"},{\"content\":{\"connectorIds\":[],\"side\":\"TOP\"},\"type\":\"ConnectorPlacement.EquallySpacedRectSide\",\"uuid\":\"fc91fa49-46f5-4ba7-960e-7bda5e0416d1\"}]},\"type\":\"ConnectorPlacement.EquallySpacedConnector\",\"uuid\":\"4bf08bc6-c7ce-47fb-af04-cd9d2b5f8092\"}],\"packageUris\":[\"http://schema.mathworks.com/mf0/Connector/19700101\"],\"version\":\"1.0\"}"
  "6.1.3.0.2 Gearbox Temperature Measurement Subsystem - O-ring " : Subsystem
      settings: PortSchema="{\"entries\":[{\"content\":{\"headerSize\":26,\"margin\":15,\"minimumSpacing\":25,\"sides\":[{\"content\":{\"connectorIds\":[]},\"type\":\"ConnectorPlacement.EquallySpacedRectSide\",\"uuid\":\"f8ee33a9-954f-44c6-a821-b5353f3278fa\"},{\"content\":{\"connectorIds\":[],\"side\":\"RIGHT\"},\"type\":\"ConnectorPlacement.EquallySpacedRectSide\",\"uuid\":\"385f1e4f-1c89-4afc-9c19-76a078cf90bc\"},{\"content\":{\"connectorIds\":[],\"side\":\"TOP\"},\"type\":\"ConnectorPlacement.EquallySpacedRectSide\",\"uuid\":\"fc91fa49-46f5-4ba7-960e-7bda5e0416d1\"}]},\"type\":\"ConnectorPlacement.EquallySpacedConnector\",\"uuid\":\"4bf08bc6-c7ce-47fb-af04-cd9d2b5f8092\"}],\"packageUris\":[\"http://schema.mathworks.com/mf0/Connector/19700101\"],\"version\":\"1.0\"}"

== system p4_system_arch_master/System 6 : Sensor and Actuation System/6.1 Sensor System /6.1.4 Gear Selection Position Measurement SubSystem  ==
  "6.1.4.1 Drum Angular Position Measurement Sensor SubSystem " : Subsystem
      settings: PortSchema="{\"entries\":[{\"content\":{\"headerSize\":26,\"margin\":15,\"minimumSpacing\":25,\"sides\":[{\"content\":{\"connectorIds\":[]},\"type\":\"ConnectorPlacement.EquallySpacedRectSide\",\"uuid\":\"f8ee33a9-954f-44c6-a821-b5353f3278fa\"},{\"content\":{\"connectorIds\":[],\"side\":\"RIGHT\"},\"type\":\"ConnectorPlacement.EquallySpacedRectSide\",\"uuid\":\"385f1e4f-1c89-4afc-9c19-76a078cf90bc\"},{\"content\":{\"connectorIds\":[],\"side\":\"TOP\"},\"type\":\"ConnectorPlacement.EquallySpacedRectSide\",\"uuid\":\"fc91fa49-46f5-4ba7-960e-7bda5e0416d1\"}]},\"type\":\"ConnectorPlacement.EquallySpacedConnector\",\"uuid\":\"4bf08bc6-c7ce-47fb-af04-cd9d2b5f8092\"}],\"packageUris\":[\"http://schema.mathworks.com/mf0/Connector/19700101\"],\"version\":\"1.0\"}"
  "6.1.4.2 Drum Angular Position Measurement Magnet SubSystem " : Subsystem
      settings: PortSchema="{\"entries\":[{\"content\":{\"headerSize\":26,\"margin\":15,\"minimumSpacing\":25,\"sides\":[{\"content\":{\"connectorIds\":[]},\"type\":\"ConnectorPlacement.EquallySpacedRectSide\",\"uuid\":\"f8ee33a9-954f-44c6-a821-b5353f3278fa\"},{\"content\":{\"connectorIds\":[],\"side\":\"RIGHT\"},\"type\":\"ConnectorPlacement.EquallySpacedRectSide\",\"uuid\":\"385f1e4f-1c89-4afc-9c19-76a078cf90bc\"},{\"content\":{\"connectorIds\":[],\"side\":\"TOP\"},\"type\":\"ConnectorPlacement.EquallySpacedRectSide\",\"uuid\":\"fc91fa49-46f5-4ba7-960e-7bda5e0416d1\"}]},\"type\":\"ConnectorPlacement.EquallySpacedConnector\",\"uuid\":\"4bf08bc6-c7ce-47fb-af04-cd9d2b5f8092\"}],\"packageUris\":[\"http://schema.mathworks.com/mf0/Connector/19700101\"],\"version\":\"1.0\"}"

== system p4_system_arch_master/System 6 : Sensor and Actuation System/6.1 Sensor System /6.1.5 Gearbox Vibration Measurement Subsystem  ==

== system p4_system_arch_master/System 6 : Sensor and Actuation System/6.1 Sensor System /6.1.6 Motor Temperature Measurement SubSystem  ==
  "6.1.6.0.1 PT100 Sensor " : Subsystem
      settings: PortSchema="{\"entries\":[{\"content\":{\"headerSize\":26,\"margin\":15,\"minimumSpacing\":25,\"sides\":[{\"content\":{\"connectorIds\":[]},\"type\":\"ConnectorPlacement.EquallySpacedRectSide\",\"uuid\":\"f8ee33a9-954f-44c6-a821-b5353f3278fa\"},{\"content\":{\"connectorIds\":[],\"side\":\"RIGHT\"},\"type\":\"ConnectorPlacement.EquallySpacedRectSide\",\"uuid\":\"385f1e4f-1c89-4afc-9c19-76a078cf90bc\"},{\"content\":{\"connectorIds\":[],\"side\":\"TOP\"},\"type\":\"ConnectorPlacement.EquallySpacedRectSide\",\"uuid\":\"fc91fa49-46f5-4ba7-960e-7bda5e0416d1\"}]},\"type\":\"ConnectorPlacement.EquallySpacedConnector\",\"uuid\":\"4bf08bc6-c7ce-47fb-af04-cd9d2b5f8092\"}],\"packageUris\":[\"http://schema.mathworks.com/mf0/Connector/19700101\"],\"version\":\"1.0\"}"

== system p4_system_arch_master/System 6 : Sensor and Actuation System/6.1 Sensor System /6.1.7 Motor Position Measurement Subsystem  ==
  "6.1.7.1 Motor Resolver - Stator Subsystem " : Subsystem
      settings: PortSchema="{\"entries\":[{\"content\":{\"headerSize\":26,\"margin\":15,\"minimumSpacing\":25,\"sides\":[{\"content\":{\"connectorIds\":[]},\"type\":\"ConnectorPlacement.EquallySpacedRectSide\",\"uuid\":\"f8ee33a9-954f-44c6-a821-b5353f3278fa\"},{\"content\":{\"connectorIds\":[],\"side\":\"RIGHT\"},\"type\":\"ConnectorPlacement.EquallySpacedRectSide\",\"uuid\":\"385f1e4f-1c89-4afc-9c19-76a078cf90bc\"},{\"content\":{\"connectorIds\":[],\"side\":\"TOP\"},\"type\":\"ConnectorPlacement.EquallySpacedRectSide\",\"uuid\":\"fc91fa49-46f5-4ba7-960e-7bda5e0416d1\"}]},\"type\":\"ConnectorPlacement.EquallySpacedConnector\",\"uuid\":\"4bf08bc6-c7ce-47fb-af04-cd9d2b5f8092\"}],\"packageUris\":[\"http://schema.mathworks.com/mf0/Connector/19700101\"],\"version\":\"1.0\"}"
  6.1.7.2 Motor Resolver - Rotor Subsystem : Subsystem
      settings: PortSchema="{\"entries\":[{\"content\":{\"headerSize\":26,\"margin\":15,\"minimumSpacing\":25,\"sides\":[{\"content\":{\"connectorIds\":[]},\"type\":\"ConnectorPlacement.EquallySpacedRectSide\",\"uuid\":\"f8ee33a9-954f-44c6-a821-b5353f3278fa\"},{\"content\":{\"connectorIds\":[],\"side\":\"RIGHT\"},\"type\":\"ConnectorPlacement.EquallySpacedRectSide\",\"uuid\":\"385f1e4f-1c89-4afc-9c19-76a078cf90bc\"},{\"content\":{\"connectorIds\":[],\"side\":\"TOP\"},\"type\":\"ConnectorPlacement.EquallySpacedRectSide\",\"uuid\":\"fc91fa49-46f5-4ba7-960e-7bda5e0416d1\"}]},\"type\":\"ConnectorPlacement.EquallySpacedConnector\",\"uuid\":\"4bf08bc6-c7ce-47fb-af04-cd9d2b5f8092\"}],\"packageUris\":[\"http://schema.mathworks.com/mf0/Connector/19700101\"],\"version\":\"1.0\"}"

== system p4_system_arch_master/System 6 : Sensor and Actuation System/6.2 Actuator System/6.2.1.0.1 Gear Selection actuator subsystem - body  ==

== system p4_system_arch_master/System 6 : Sensor and Actuation System/6.2 Actuator System/6.2.1.0.2 Gear Selection actuator subsystem - Shaft ==
